simulink model "sf_sawtooth1_2018a"  (R2018a)
settings: Solver=VariableStepAuto  StartTime=0.0  StopTime=10.0  RelTol=1e-3
settings Model: Creator=bzhan  LastModifiedBy=bzhan
settings DataIOCC: ReturnWorkspaceOutputs=on
settings SFSimCC: SimUseLocalCustomCode=on
settings RTWCC: RTWUseLocalCustomCode=on

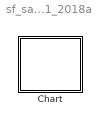
== system sf_sawtooth1_2018a ==
  Chart : Stateflow chart  TreatAsAtomicUnit=on

== stateflow chart sf_sawtooth1_2018a/Chart ==
  settings: updateMethod=CONTINUOUS
  state A
    du: x_dot=1; t_dot=1;
  (default) -> A : {t=0;x=0}
  A -> A : [t>=1]{t=0;x=0;}
  data: t local; x local
  data t settings: updateMethod=SF_CONTINUOUS_TIME_DATA
  data x settings: updateMethod=SF_CONTINUOUS_TIME_DATA
